simulink model "inverse_kinematic_controller_1"  (R2019b)
settings: Solver=FixedStepAuto  StartTime=0.0  StopTime=250  FixedStep=0.01  RelTol=1e-3
values from neighbouring files (symbols this model uses):
  px = px/100    [path_gen.m]
  py = 0.5*sin(px)    [path_gen.m]
libraries: simulink x1
settings Model: Creator=ASUS  LastModifiedBy=ASUS
settings DataIOCC: ReturnWorkspaceOutputs=off

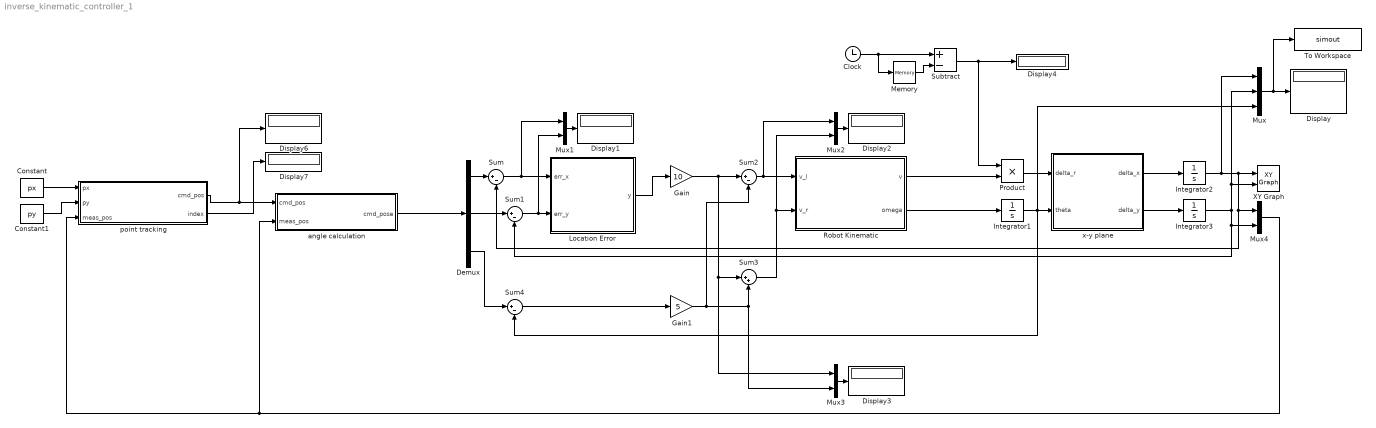
== system inverse_kinematic_controller_1 ==
  Clock : Clock
  Constant : Constant  Value=px
  Constant1 : Constant  Value=py
  Demux : Demux  Outputs=3
  Display{,1..4,6..7} (7 alike) : Display
  Gain : Gain  Gain=10
  Gain1 : Gain  Gain=5
  Integrator1 : Integrator
  Integrator2 : Integrator
  Integrator3 : Integrator
  Location Error : MATLAB Function  TreatAsAtomicUnit=on
  Memory : Memory
  Mux : Mux  Inputs=3
  Mux{1..4} (4 alike) : Mux  Inputs=2
  Product : Product
  Robot Kinematic : MATLAB Function  TreatAsAtomicUnit=on
  Subtract : Sum  Inputs=+-
  Sum{,1..2,4} (4 alike) : Sum  Inputs=|+-
  Sum3 : Sum  Inputs=|++
  To Workspace : ToWorkspace  VariableName=simout  SaveFormat=Timeseries  SampleTime=-1
  XY Graph : simulink/Sinks/XY Graph  xmin=-5  xmax=5  ymin=-5  ymax=5  st=-1
  angle calculation : MATLAB Function  TreatAsAtomicUnit=on
  point tracking : MATLAB Function  TreatAsAtomicUnit=on
  x-y plane : MATLAB Function  TreatAsAtomicUnit=on
  wires:
  Robot Kinematic/1(v) -> Product/2
  Robot Kinematic/2(omega) -> Integrator1/1
  Integrator1/1 -> Sum4/2, Mux/3, x-y plane/2(theta)
  Product/1 -> x-y plane/1(delta_r)
  x-y plane/1(delta_x) -> Integrator2/1
  x-y plane/2(delta_y) -> Integrator3/1
  Integrator2/1 -> Mux/1, XY Graph/1, Mux4/1, Sum/2
  Integrator3/1 -> Mux/2, XY Graph/2, Sum1/2, Mux4/2
  Demux/1 -> Sum/1
  Demux/2 -> Sum1/1
  Sum/1 -> Mux1/1, Location Error/1(err_x)
  Sum1/1 -> Mux1/2, Location Error/2(err_y)
  Location Error/1(y) -> Gain/1
  Gain/1 -> Mux3/1, Sum3/1, Sum2/1
  Sum2/1 -> Mux2/1, Robot Kinematic/1(v_l)
  Gain1/1 -> Sum2/2, Mux3/2, Sum3/2
  Sum3/1 -> Mux2/2, Robot Kinematic/2(v_r)
  Demux/3 -> Sum4/1
  Sum4/1 -> Gain1/1
  Mux/1 -> To Workspace/1, Display/1
  Mux1/1 -> Display1/1
  Mux2/1 -> Display2/1
  Mux3/1 -> Display3/1
  Mux4/1 -> angle calculation/2(meas_pos), point tracking/3(meas_pos)
  angle calculation/1(cmd_pose) -> Demux/1
  Constant/1 -> point tracking/1(px)
  point tracking/1(cmd_pos) -> Display6/1, angle calculation/1(cmd_pos)
  Memory/1 -> Subtract/2
  Clock/1 -> Subtract/1, Memory/1
  Subtract/1 -> Display4/1, Product/1
  Constant1/1 -> point tracking/2(py)
  point tracking/2(index) -> Display7/1

== matlab function inverse_kinematic_controller_1/x-y plane ==
  data: delta_x output; delta_y output; delta_r input; theta input
function [delta_x,delta_y] = xy_plane(delta_r,theta)

delta_x = delta_r*cos(theta);
delta_y = delta_r*sin(theta);

== matlab function inverse_kinematic_controller_1/Robot Kinematic ==
  data: v output; v_l input; v_r input; omega output
function [v,omega] = robot_kinematic(v_l,v_r)

d = 0.34;

v = (v_r + v_l)/2;
omega = (v_r - v_l)/d;

== matlab function inverse_kinematic_controller_1/Location Error ==
  data: err_x input; y output; err_y input
function y = location_err(err_x,err_y)

y = sqrt(err_x^2+err_y^2);

== matlab function inverse_kinematic_controller_1/angle calculation ==
  data: cmd_pos input; cmd_pose output; meas_pos input
function cmd_pose = angle_cal(cmd_pos,meas_pos)

cmd_angle = atan( (cmd_pos(2)-meas_pos(2)) / (cmd_pos(1)-meas_pos(1)));

cmd_pose = [cmd_pos(1) cmd_pos(2) cmd_angle];

== matlab function inverse_kinematic_controller_1/point tracking ==
  settings: updateMethod=DISCRETE
  data: px input; py input; cmd_pos output; meas_pos input; index output
function [cmd_pos,index] = point_tracking(px,py,meas_pos)

% Run path_gen.m first to generate path

point_tolerance = 0.01;

% index of waypoints
persistent i;
if isempty(i)
    i=1;
end

if (abs(meas_pos(1) - px(i)) < point_tolerance) && (abs(meas_pos(2) - py(i)) < point_tolerance)
    if i < size(px,1)
        i = i + 1;
    end
end
index = i;
cmd_pos = [px(i) py(i)];
